simulink model "code_gen_man_bin"  (Simulink 7.5)
settings: Solver=FixedStepDiscrete  SolverMode=SingleTasking  StartTime=0.0  StopTime=10.0  FixedStep=0.01  RelTol=1e-3
InitFcn:
  | boat_constants
values from neighbouring files (symbols this model uses):
  figure8_waypoints = int32([ ... (first row only)    [boat_constants.m]
  InitialPoint = 0    [boat_constants.m]    (also in l2plus.m)
  IPStar = 0    [boat_constants.m]    (also in l2plus.m)
  ISA_g = 9.815    [boat_constants.m]
  MaxDwnPthStar = 1    [boat_constants.m]    (also in l2plus.m)
  OC2max = 49999    [boat_constants.m]    (also in simulation_constants.m)
  sampling_waypoints = int32([ ... (first row only)    [boat_constants.m]
  switchDistance = 4    [boat_constants.m]    (also in l2plus.m)
  T_step = 0.01    [boat_constants.m]    (also in common.m)
  tanIntercept = tan( 45*pi/180 )    [boat_constants.m]    (also in l2plus.m)
  test_waypoints = int32([ ... (first row only)    [boat_constants.m]
  TStar = single(4.5)    [boat_constants.m]    (also in l2plus.m = single(2))
  Turn2Track = 0    [boat_constants.m]    (also in l2plus.m)
  wheelbase = 3.27    [boat_constants.m]
undefined symbols (not defined in the file or in its folder): clearGpsData, clearSensorData, cpInitCommunications, DataEEInitAndClear, DataEEWrite, DiscIntNeverNeededParam, ecan1_buffered_transmit_matlab, ecan1_error_status_matlab, ecan1_init, GetAirData, getGpsData, getRevoData, getSensorData, GetThrottleData, GetWaterData, GetWindData, Init_onlyOnce, Init_Reset, initCalibrationRange, initGps, processNewCommData, processNewGpsData, processNewRevoData, setHilMode, u1, u2, uart1EnqueueStateData, uart2EnqueueActuatorData, y1
libraries: simulink x80, dsPICdrivers x50, uSimLib x4, simulink_need_slupdate x4
(part 5 of 6)

== system code_gen_man_bin/Controller/Radio Control Inputs1/Calibration/Update range from input1 ==
  note: Update lower range limit.
      | The new value is checked against a sane range of 5000-11000
      | to keep values realistic.
  note: Update upper range limit
  limitRange : Inport
  newValue : Inport  Port=2
  If : If  NumInputs=2  IfExpression=u1 < u2 & u1 > 5000 & u1 >= 0
  If Action Subsystem : Subsystem  TreatAsAtomicUnit=on
  If Action Subsystem1 : Subsystem  TreatAsAtomicUnit=on
  If Action Subsystem2 : Subsystem  TreatAsAtomicUnit=on
  If Action Subsystem3 : Subsystem  TreatAsAtomicUnit=on
  If1 : If  NumInputs=2  IfExpression=u1 > u2 & u1 < 11000 & u1 >= 0
  Merge : Merge
  Merge1 : Merge
  Mux : Mux  Inputs=2
  Selector : Selector  InputPortWidth=2  IndexOptions=Index vector (dialog)  Indices=[1]  OutputSizes=1
  Selector1 : Selector  InputPortWidth=2  IndexOptions=Index vector (dialog)  Indices=[2]  OutputSizes=1
  newRange : Outport
  wires:
  Selector/1 -> If/2, If Action Subsystem1/1(In1)
  Selector1/1 -> If Action Subsystem3/1(In1), If1/2
  Mux/1 -> newRange/1
  Merge1/1 -> Mux/2
  Merge/1 -> Mux/1
  If Action Subsystem3/1(Out1) -> Merge1/2
  If Action Subsystem2/1(Out1) -> Merge1/1
  If1/2 -> If Action Subsystem3/Action
  If1/1 -> If Action Subsystem2/Action
  If Action Subsystem1/1(Out1) -> Merge/2
  If Action Subsystem/1(Out1) -> Merge/1
  If/2 -> If Action Subsystem1/Action
  If/1 -> If Action Subsystem/Action
  newValue/1 -> If Action Subsystem/1(In1), If/1, If Action Subsystem2/1(In1), If1/1
  limitRange/1 -> Selector/1, Selector1/1

== system code_gen_man_bin/Controller/Radio Control Inputs1/Calibration/Update range from input2 ==
  note: Update lower range limit.
      | The new value is checked against a sane range of 5000-11000
      | to keep values realistic.
  note: Update upper range limit
  limitRange : Inport
  newValue : Inport  Port=2
  If : If  NumInputs=2  IfExpression=u1 < u2 & u1 > 5000 & u1 >= 0
  If Action Subsystem : Subsystem  TreatAsAtomicUnit=on
  If Action Subsystem1 : Subsystem  TreatAsAtomicUnit=on
  If Action Subsystem2 : Subsystem  TreatAsAtomicUnit=on
  If Action Subsystem3 : Subsystem  TreatAsAtomicUnit=on
  If1 : If  NumInputs=2  IfExpression=u1 > u2 & u1 < 11000 & u1 >= 0
  Merge : Merge
  Merge1 : Merge
  Mux : Mux  Inputs=2
  Selector : Selector  InputPortWidth=2  IndexOptions=Index vector (dialog)  Indices=[1]  OutputSizes=1
  Selector1 : Selector  InputPortWidth=2  IndexOptions=Index vector (dialog)  Indices=[2]  OutputSizes=1
  newRange : Outport
  wires:
  Selector/1 -> If/2, If Action Subsystem1/1(In1)
  Selector1/1 -> If Action Subsystem3/1(In1), If1/2
  Mux/1 -> newRange/1
  Merge1/1 -> Mux/2
  Merge/1 -> Mux/1
  If Action Subsystem3/1(Out1) -> Merge1/2
  If Action Subsystem2/1(Out1) -> Merge1/1
  If1/2 -> If Action Subsystem3/Action
  If1/1 -> If Action Subsystem2/Action
  If Action Subsystem1/1(Out1) -> Merge/2
  If Action Subsystem/1(Out1) -> Merge/1
  If/2 -> If Action Subsystem1/Action
  If/1 -> If Action Subsystem/Action
  newValue/1 -> If Action Subsystem/1(In1), If/1, If Action Subsystem2/1(In1), If1/1
  limitRange/1 -> Selector/1, Selector1/1

== system code_gen_man_bin/Controller/Radio Control Inputs1/Detect calibration trigger/State outputs ==
  note: Define state outputs:
      | State 0: Not in calibration mode
      |   - LED is off
      | State 1: Calibration mode trigger test
      |   - LED is blinking at 10Hz
      | State 2: Calibration mode
      |   - LED is on
  cState : Inport
  If Action Subsystem1 : Subsystem  TreatAsAtomicUnit=on
  If Action Subsystem2 : Subsystem  TreatAsAtomicUnit=on
  If Action Subsystem3 : Subsystem  TreatAsAtomicUnit=on
  If Action Subsystem4 : Subsystem  TreatAsAtomicUnit=on
  If1 : If  IfExpression=u1 == 0 | u1 == 3  ElseIfExpressions=u1 == 1 | u1 == 4, u1 == 2
  Merge : Merge  Inputs=4  InitialOutput=false
  Rate Transition : RateTransition
  Repeating Sequence Stair : simulink/Sources/Repeating Sequence Stair  SystemSampleTime=-1  OutValues=[1 0]  tsamp=.1  OutMin=[]  OutMax=[]  OutDataTypeStr=fixdt('boolean')  OutputDataTypeScalingMode=Specify via dialog  OutDataType=fixdt('boolean')  ConRadixGroup=Best Precision: Vector-wise  OutScaling=[]
  LED : Outport
  wires:
  cState/1 -> If1/1
  Merge/1 -> LED/1
  If1/1 -> If Action Subsystem1/Action
  If1/2 -> If Action Subsystem3/Action
  If Action Subsystem1/1(LED) -> Merge/1
  If Action Subsystem3/1(LED) -> Merge/2
  If1/4 -> If Action Subsystem2/Action
  If1/3 -> If Action Subsystem4/Action
  If Action Subsystem4/1(LED) -> Merge/3
  If Action Subsystem2/1(LED) -> Merge/4
  Repeating Sequence Stair/1 -> Rate Transition/1
  Rate Transition/1 -> If Action Subsystem3/1(Pulse)

== system code_gen_man_bin/Controller/Radio Control Inputs1/If Action Subsystem1/Add 8% center deadband ==
  In1 : Inport
  If : If  IfExpression=u1 > -36 & u1 < 36
  If Action Subsystem : Subsystem  TreatAsAtomicUnit=on
  If Action Subsystem1 : Subsystem  TreatAsAtomicUnit=on
  Merge : Merge
  Out1 : Outport
  wires:
  In1/1 -> If Action Subsystem/1(In1), If/1
  If/2 -> If Action Subsystem/Action
  If/1 -> If Action Subsystem1/Action
  If Action Subsystem/1(Out1) -> Merge/2
  If Action Subsystem1/1(Out1) -> Merge/1
  Merge/1 -> Out1/1

== system code_gen_man_bin/Controller/Radio Control Inputs1/If Action Subsystem3/Add 5% deadband about 0 ==
  In1 : Inport
  If : If  IfExpression=u1 < 43 & u1 > -43
  If Action Subsystem : Subsystem  TreatAsAtomicUnit=on
  If Action Subsystem1 : Subsystem  TreatAsAtomicUnit=on
  Merge : Merge
  Out1 : Outport
  wires:
  In1/1 -> If Action Subsystem/1(In1), If/1
  If/2 -> If Action Subsystem/Action
  If/1 -> If Action Subsystem1/Action
  If Action Subsystem1/1(Out1) -> Merge/1
  Merge/1 -> Out1/1
  If Action Subsystem/1(Out1) -> Merge/2

== system code_gen_man_bin/Controller/Radio Control Inputs1/If Action Subsystem5/Add 8% center deadband ==
  In1 : Inport
  If : If  IfExpression=u1 > 460 & u1 < 540
  If Action Subsystem : Subsystem  TreatAsAtomicUnit=on
  If Action Subsystem1 : Subsystem  TreatAsAtomicUnit=on
  Merge : Merge
  Out1 : Outport
  wires:
  In1/1 -> If Action Subsystem/1(In1), If/1
  If/2 -> If Action Subsystem/Action
  If/1 -> If Action Subsystem1/Action
  If Action Subsystem/1(Out1) -> Merge/2
  If Action Subsystem1/1(Out1) -> Merge/1
  Merge/1 -> Out1/1

== system code_gen_man_bin/Controller/Rudder sensor calibration/Throttle Command/Mux Everything ==
  reset : Inport  OutDataType=sfix(16)  OutScaling=2^0
  0x300 : Constant  Value=768  OutDataTypeMode=uint32  OutDataType=sfix(16)  OutScaling=2^0  OutDataTypeStr=uint32
  Data Type Conversion1 : DataTypeConversion  OutDataTypeMode=boolean  OutDataType=sfix(16)  OutScaling=2^0  OutDataTypeStr=boolean
  Data Type Conversion3 : DataTypeConversion  OutDataTypeMode=boolean  OutDataType=sfix(16)  OutScaling=2^0  OutDataTypeStr=boolean
  Detect Change : simulink/Logic and Bit Operations/Detect Change  SystemSampleTime=-1  vinit=0
  Detect Rise Positive : simulink/Logic and Bit Operations/Detect Rise Positive  SystemSampleTime=-1  vinit=0
  Disable motor : Constant  Value=[0 0 0 0 64 0]  OutDataTypeMode=uint8  OutDataType=sfix(16)  OutScaling=2^0  OutDataTypeStr=uint8
  Enable motor : Constant  Value=[0 0 0 0 32 0]  OutDataTypeMode=uint8  OutDataType=sfix(16)  OutScaling=2^0  OutDataTypeStr=uint8
  Message Length1 : Probe  ProbeSampleTime=off  ProbeComplexSignal=off  ProbeWidthDataType=uint8
  Switch : Switch  Criteria=u2 ~= 0  OutDataType=fixdt(1, 16)  OutScaling=2^0
  iden : Outport  OutDataType=sfix(16)  OutScaling=2^0
  data : Outport  Port=2  OutDataType=sfix(16)  OutScaling=2^0
  size : Outport  Port=3  OutDataType=sfix(16)  OutScaling=2^0
  trig : Outport  Port=4  OutDataType=sfix(16)  OutScaling=2^0
  wires:
  0x300/1 -> iden/1
  Message Length1/1 -> size/1
  Switch/1 -> data/1, Message Length1/1
  Disable motor/1 -> Switch/1
  Enable motor/1 -> Switch/3
  Data Type Conversion1/1 -> Switch/2
  Detect Rise Positive/1 -> Data Type Conversion1/1
  reset/1 -> Detect Rise Positive/1, Detect Change/1
  Detect Change/1 -> Data Type Conversion3/1
  Data Type Conversion3/1 -> trig/1

== system code_gen_man_bin/Controller/Split trackCommand to singular commands/Countdown timer for trigger/State transitions ==
  note: Define state transitions:
      | State 0: Not in calibration mode
      |   - Transition to state 1 if change
      | State 1: Transition trigger test
      |   - Transition to state 2 if level held
      |   - Transition to state 0 if level drops
      | State 2: Transition successful
      |   - Transition to state 0 if change
  timer : Inport
  level : Inport  Port=2
  timerState : Inport  Port=3
  If : If  NumInputs=3  IfExpression=u3 == 0 & u2 == 1  ElseIfExpressions=u3 == 1 & u2 == 0, u3 == 1 & u1 >= 100, u3 == 2 & u2 == 0
  Merge1 : Merge  Inputs=5  InitialOutput=false
  Merge2 : Merge  Inputs=5  InitialOutput=false
  Null transition (necessary for merge block) : Subsystem  TreatAsAtomicUnit=on
  Transition from 0 to 1 : Subsystem  TreatAsAtomicUnit=on
  Transition from 1 to 0 : Subsystem  TreatAsAtomicUnit=on
  Transition from 1 to 2 : Subsystem  TreatAsAtomicUnit=on
  Transition from 2 to 0 : Subsystem  TreatAsAtomicUnit=on
  startTimer : Outport
  trigger : Outport  Port=2
  wires:
  If/1 -> Transition from 0 to 1/Action
  If/5 -> Null transition (necessary for merge block)/Action
  timer/1 -> If/1
  timerState/1 -> If/3
  level/1 -> If/2
  If/2 -> Transition from 1 to 0/Action
  If/3 -> Transition from 1 to 2/Action
  If/4 -> Transition from 2 to 0/Action
  Merge1/1 -> startTimer/1
  Transition from 0 to 1/1(startTimer) -> Merge1/1
  Transition from 1 to 0/1(startTimer) -> Merge1/2
  Transition from 1 to 2/1(startTimer) -> Merge1/3
  Transition from 2 to 0/1(startTimer) -> Merge1/4
  Null transition (necessary for merge block)/1(startTimer) -> Merge1/5
  Merge2/1 -> trigger/1
  Transition from 0 to 1/2(trigger) -> Merge2/1
  Transition from 1 to 0/2(trigger) -> Merge2/2
  Transition from 1 to 2/2(trigger) -> Merge2/3
  Transition from 2 to 0/2(trigger) -> Merge2/4
  Null transition (necessary for merge block)/2(trigger) -> Merge2/5

== system code_gen_man_bin/Controller/Split trackCommand to singular commands/Countdown timer for trigger1/State transitions ==
  note: Define state transitions:
      | State 0: Not in calibration mode
      |   - Transition to state 1 if change
      | State 1: Transition trigger test
      |   - Transition to state 2 if level held
      |   - Transition to state 0 if level drops
      | State 2: Transition successful
      |   - Transition to state 0 if change
  timer : Inport
  level : Inport  Port=2
  timerState : Inport  Port=3
  If : If  NumInputs=3  IfExpression=u3 == 0 & u2 == 1  ElseIfExpressions=u3 == 1 & u2 == 0, u3 == 1 & u1 >= 100, u3 == 2 & u2 == 0
  Merge1 : Merge  Inputs=5  InitialOutput=false
  Merge2 : Merge  Inputs=5  InitialOutput=false
  Null transition (necessary for merge block) : Subsystem  TreatAsAtomicUnit=on
  Transition from 0 to 1 : Subsystem  TreatAsAtomicUnit=on
  Transition from 1 to 0 : Subsystem  TreatAsAtomicUnit=on
  Transition from 1 to 2 : Subsystem  TreatAsAtomicUnit=on
  Transition from 2 to 0 : Subsystem  TreatAsAtomicUnit=on
  startTimer : Outport
  trigger : Outport  Port=2
  wires:
  Null transition (necessary for merge block)/2(trigger) -> Merge2/5
  Transition from 2 to 0/2(trigger) -> Merge2/4
  Transition from 1 to 2/2(trigger) -> Merge2/3
  Transition from 1 to 0/2(trigger) -> Merge2/2
  Transition from 0 to 1/2(trigger) -> Merge2/1
  Merge2/1 -> trigger/1
  Null transition (necessary for merge block)/1(startTimer) -> Merge1/5
  Transition from 2 to 0/1(startTimer) -> Merge1/4
  Transition from 1 to 2/1(startTimer) -> Merge1/3
  Transition from 1 to 0/1(startTimer) -> Merge1/2
  Transition from 0 to 1/1(startTimer) -> Merge1/1
  Merge1/1 -> startTimer/1
  If/4 -> Transition from 2 to 0/Action
  If/3 -> Transition from 1 to 2/Action
  If/2 -> Transition from 1 to 0/Action
  level/1 -> If/2
  timerState/1 -> If/3
  timer/1 -> If/1
  If/5 -> Null transition (necessary for merge block)/Action
  If/1 -> Transition from 0 to 1/Action

== system code_gen_man_bin/Controller/Autonomous Controller/State Keeper & Estimator/GPS Estimator/Subsystem ==
  note: Multiply by .51444 to
      | convert knots to m/s
  gps : Inport
  Angle Conversion : uSimLib/Conversions/Angle Conversion  SystemSampleTime=-1  iu=deg  ou=rad
  Bus Selector : BusSelector  OutputSignals=sog
  Bus Selector1 : BusSelector  OutputSignals=cog
  Constant : Constant  Value=0  OutDataTypeMode=single  OutDataType=fixdt(1, 16)  OutScaling=2^0  OutDataTypeStr=single
  Gain : Gain  Gain=.5144444  ParameterDataType=fixdt(1, 16)  ParameterScaling=2^0  OutDataType=fixdt(1, 16)  OutScaling=2^0
  Mux : Mux  Inputs=3
  Product : Product  OutDataTypeMode=single  OutDataType=fixdt(1, 16)  OutScaling=2^0  OutDataTypeStr=single  RndMeth=Zero
  Product1 : Product  OutDataTypeMode=single  OutDataType=fixdt(1, 16)  OutScaling=2^0  OutDataTypeStr=single  RndMeth=Zero
  Reorder : Subsystem
  Trigonometric Function : Trigonometry
  Trigonometric Function1 : Trigonometry  Operator=cos
  velocity : Outport
  heading : Outport  Port=2
  pos : Outport  Port=3
  time : Outport  Port=4
  wires:
  Reorder/2(time) -> time/1
  Reorder/1(pos) -> pos/1
  Bus Selector/1 -> Gain/1  "<sog>"
  Angle Conversion/1 -> Trigonometric Function1/1, Trigonometric Function/1, heading/1
  Mux/1 -> velocity/1
  Constant/1 -> Mux/3
  Product/1 -> Mux/2
  Product1/1 -> Mux/1
  Trigonometric Function1/1 -> Product1/2
  Trigonometric Function/1 -> Product/2
  Bus Selector1/1 -> Angle Conversion/1  "<cog>"
  gps/1 -> Bus Selector1/1, Bus Selector/1, Reorder/1(In1)
  Gain/1 -> Product/1, Product1/1

== system code_gen_man_bin/Controller/Autonomous Controller/Throttle Command/Mux Everything/Build speed command ==
  CC : Inport  OutDataType=sfix(16)  OutScaling=2^0
  Constant : Constant  OutDataTypeMode=uint8  OutDataType=sfix(16)  OutScaling=2^0  OutDataTypeStr=uint8
  Constant1 : Constant  Value=0  OutDataTypeMode=uint8  OutDataType=sfix(16)  OutScaling=2^0  OutDataTypeStr=uint8
  Constant2 : Constant  Value=0  OutDataTypeMode=uint8  OutDataType=sfix(16)  OutScaling=2^0  OutDataTypeStr=uint8
  Constant3 : Constant  Value=5  OutDataTypeMode=uint8  OutDataType=sfix(16)  OutScaling=2^0  OutDataTypeStr=uint8
  Mux : Mux  Inputs=5
  uint16 to uchar : Subsystem  AncestorBlock=uSimLib/Conversions/uint16 to uchar
  msg : Outport  OutDataType=sfix(16)  OutScaling=2^0
  wires:
  CC/1 -> uint16 to uchar/1(ushort)
  Constant2/1 -> Mux/5
  Constant1/1 -> Mux/4
  Mux/1 -> msg/1
  Constant3/1 -> Mux/2
  Constant/1 -> Mux/1
  uint16 to uchar/1(uchar) -> Mux/3

== system code_gen_man_bin/Controller/RC Inputs/Map PWM values to Actuator Signals/Throttle Command/Mux Everything ==
  speed : Inport  OutDataType=sfix(16)  OutScaling=2^0
  enable : Inport  Port=2  OutDataType=sfix(16)  OutScaling=2^0
  Throttle : Inport  Port=3  OutDataType=sfix(16)  OutScaling=2^0
  0x300 : Constant  Value=768  OutDataTypeMode=uint32  OutDataType=sfix(16)  OutScaling=2^0  OutDataTypeStr=uint32
  0x301 : Constant  Value=769  OutDataTypeMode=uint32  OutDataType=sfix(16)  OutScaling=2^0  OutDataTypeStr=uint32
  Build speed command : Subsystem
  Enable motor : Constant  Value=[0 0 0 0 32 0]  OutDataTypeMode=uint8  OutDataType=sfix(16)  OutScaling=2^0  OutDataTypeStr=uint8
  Message Length1 : Probe  ProbeSampleTime=off  ProbeComplexSignal=off  ProbeWidthDataType=uint8
  Switch : Switch  Criteria=u2 ~= 0  Threshold=1
  Switch1 : Switch  Criteria=u2 ~= 0  OutDataType=fixdt(1, 16)  OutScaling=2^0
  iden : Outport  OutDataType=sfix(16)  OutScaling=2^0
  data : Outport  Port=2  OutDataType=sfix(16)  OutScaling=2^0
  size : Outport  Port=3  OutDataType=sfix(16)  OutScaling=2^0
  trig : Outport  Port=4  OutDataType=sfix(16)  OutScaling=2^0
  wires:
  Throttle/1 -> Build speed command/1(CC)
  Message Length1/1 -> size/1
  0x301/1 -> Switch/3
  Switch1/1 -> Message Length1/1, data/1
  0x300/1 -> Switch/1
  enable/1 -> Switch/2, Switch1/2
  speed/1 -> trig/1
  Enable motor/1 -> Switch1/1
  Build speed command/1(msg) -> Switch1/3
  Switch/1 -> iden/1

== system code_gen_man_bin/Controller/RC Inputs/Map PWM values to Actuator Signals/Throttle Command/Trigger Events ==
  Throttle : Inport  OutDataType=sfix(16)  OutScaling=2^0
  Data Type Conversion3 : DataTypeConversion  OutDataTypeMode=boolean  OutDataType=sfix(16)  OutScaling=2^0  OutDataTypeStr=boolean
  Detect Change : simulink/Logic and Bit Operations/Detect Change  SystemSampleTime=-1  vinit=0
  Shift Arithmetic : simulink/Logic and Bit Operations/Shift Arithmetic  SystemSampleTime=-1  nBitShiftRight=2  nBinPtShiftRight=0
  Weighted Moving Average : simulink_need_slupdate/Weighted Moving Average  mgainval=[.5 .5]  vinit=0.0  samptime=-1  OutDataTypeStr=Inherit: Inherit via back propagation  OutDataType=sfix(16)  OutScaling=2^-10  DoSatur=off  GainDataType=uint(16)  MatRadixGroup=Best Precision: Matrix-wise  GainScaling=2^-10
  Change Speed : Outport  OutDataType=sfix(16)  OutScaling=2^0
  wires:
  Throttle/1 -> Shift Arithmetic/1
  Detect Change/1 -> Data Type Conversion3/1
  Data Type Conversion3/1 -> Change Speed/1
  Weighted Moving Average/1 -> Detect Change/1
  Shift Arithmetic/1 -> Weighted Moving Average/1

== system code_gen_man_bin/Controller/Radio Control Inputs1/Calibration/Update range from input/If Action Subsystem ==
  In1 : Inport  OutDataType=fixdt(1, 16)  OutScaling=2^0
  Action Port : ActionPort  ActionType=then
  Out1 : Outport  OutDataType=fixdt(1, 16)  OutScaling=2^0
  wires:
  In1/1 -> Out1/1

== system code_gen_man_bin/Controller/Radio Control Inputs1/Calibration/Update range from input/If Action Subsystem1 ==
  In1 : Inport  OutDataType=fixdt(1, 16)  OutScaling=2^0
  Action Port : ActionPort  ActionType=else
  Out1 : Outport  OutDataType=fixdt(1, 16)  OutScaling=2^0
  wires:
  In1/1 -> Out1/1

== system code_gen_man_bin/Controller/Radio Control Inputs1/Calibration/Update range from input/If Action Subsystem2 ==
  In1 : Inport  OutDataType=fixdt(1, 16)  OutScaling=2^0
  Action Port : ActionPort  ActionType=then
  Out1 : Outport  OutDataType=fixdt(1, 16)  OutScaling=2^0
  wires:
  In1/1 -> Out1/1

== system code_gen_man_bin/Controller/Radio Control Inputs1/Calibration/Update range from input/If Action Subsystem3 ==
  In1 : Inport  OutDataType=fixdt(1, 16)  OutScaling=2^0
  Action Port : ActionPort  ActionType=else
  Out1 : Outport  OutDataType=fixdt(1, 16)  OutScaling=2^0
  wires:
  In1/1 -> Out1/1

== system code_gen_man_bin/Controller/Radio Control Inputs1/Calibration/Update range from input1/If Action Subsystem ==
  In1 : Inport  OutDataType=fixdt(1, 16)  OutScaling=2^0
  Action Port : ActionPort  ActionType=then
  Out1 : Outport  OutDataType=fixdt(1, 16)  OutScaling=2^0
  wires:
  In1/1 -> Out1/1

== system code_gen_man_bin/Controller/Radio Control Inputs1/Calibration/Update range from input1/If Action Subsystem1 ==
  In1 : Inport  OutDataType=fixdt(1, 16)  OutScaling=2^0
  Action Port : ActionPort  ActionType=else
  Out1 : Outport  OutDataType=fixdt(1, 16)  OutScaling=2^0
  wires:
  In1/1 -> Out1/1

== system code_gen_man_bin/Controller/Radio Control Inputs1/Calibration/Update range from input1/If Action Subsystem2 ==
  In1 : Inport  OutDataType=fixdt(1, 16)  OutScaling=2^0
  Action Port : ActionPort  ActionType=then
  Out1 : Outport  OutDataType=fixdt(1, 16)  OutScaling=2^0
  wires:
  In1/1 -> Out1/1

== system code_gen_man_bin/Controller/Radio Control Inputs1/Calibration/Update range from input1/If Action Subsystem3 ==
  In1 : Inport  OutDataType=fixdt(1, 16)  OutScaling=2^0
  Action Port : ActionPort  ActionType=else
  Out1 : Outport  OutDataType=fixdt(1, 16)  OutScaling=2^0
  wires:
  In1/1 -> Out1/1

== system code_gen_man_bin/Controller/Radio Control Inputs1/Calibration/Update range from input2/If Action Subsystem ==
  In1 : Inport  OutDataType=fixdt(1, 16)  OutScaling=2^0
  Action Port : ActionPort  ActionType=then
  Out1 : Outport  OutDataType=fixdt(1, 16)  OutScaling=2^0
  wires:
  In1/1 -> Out1/1

== system code_gen_man_bin/Controller/Radio Control Inputs1/Calibration/Update range from input2/If Action Subsystem1 ==
  In1 : Inport  OutDataType=fixdt(1, 16)  OutScaling=2^0
  Action Port : ActionPort  ActionType=else
  Out1 : Outport  OutDataType=fixdt(1, 16)  OutScaling=2^0
  wires:
  In1/1 -> Out1/1

== system code_gen_man_bin/Controller/Radio Control Inputs1/Calibration/Update range from input2/If Action Subsystem2 ==
  In1 : Inport  OutDataType=fixdt(1, 16)  OutScaling=2^0
  Action Port : ActionPort  ActionType=then
  Out1 : Outport  OutDataType=fixdt(1, 16)  OutScaling=2^0
  wires:
  In1/1 -> Out1/1

== system code_gen_man_bin/Controller/Radio Control Inputs1/Calibration/Update range from input2/If Action Subsystem3 ==
  In1 : Inport  OutDataType=fixdt(1, 16)  OutScaling=2^0
  Action Port : ActionPort  ActionType=else
  Out1 : Outport  OutDataType=fixdt(1, 16)  OutScaling=2^0
  wires:
  In1/1 -> Out1/1

== system code_gen_man_bin/Controller/Radio Control Inputs1/Detect calibration trigger/State outputs/If Action Subsystem1 ==
  Action Port : ActionPort  ActionType=then
  Constant1 : Constant  Value=false  OutDataType=fixdt(1, 16)  OutScaling=2^0  OutDataTypeStr=Inherit: Inherit via back propagation
  LED : Outport  OutDataType=fixdt(1, 16)  OutScaling=2^0  InitialOutput=false
  wires:
  Constant1/1 -> LED/1

== system code_gen_man_bin/Controller/Radio Control Inputs1/Detect calibration trigger/State outputs/If Action Subsystem2 ==
  Action Port : ActionPort  ActionType=else
  Constant1 : Constant  Value=false  OutDataType=fixdt(1, 16)  OutScaling=2^0  OutDataTypeStr=Inherit: Inherit via back propagation
  LED : Outport  OutDataType=fixdt(1, 16)  OutScaling=2^0  InitialOutput=false
  wires:
  Constant1/1 -> LED/1

== system code_gen_man_bin/Controller/Radio Control Inputs1/Detect calibration trigger/State outputs/If Action Subsystem3 ==
  Pulse : Inport
  Action Port : ActionPort  ActionType=elseif
  LED : Outport  OutDataType=fixdt(1, 16)  OutScaling=2^0  InitialOutput=false
  wires:
  Pulse/1 -> LED/1

== system code_gen_man_bin/Controller/Radio Control Inputs1/Detect calibration trigger/State outputs/If Action Subsystem4 ==
  Action Port : ActionPort  ActionType=elseif
  Constant1 : Constant  Value=true  OutDataType=fixdt(1, 16)  OutScaling=2^0  OutDataTypeStr=Inherit: Inherit via back propagation
  LED : Outport  OutDataType=fixdt(1, 16)  OutScaling=2^0  InitialOutput=false
  wires:
  Constant1/1 -> LED/1

== system code_gen_man_bin/Controller/Radio Control Inputs1/If Action Subsystem1/Add 8% center deadband/If Action Subsystem ==
  In1 : Inport  OutDataType=fixdt(1, 16)  OutScaling=2^0
  Action Port : ActionPort  ActionType=else
  Out1 : Outport  OutDataType=fixdt(1, 16)  OutScaling=2^0
  wires:
  In1/1 -> Out1/1

== system code_gen_man_bin/Controller/Radio Control Inputs1/If Action Subsystem1/Add 8% center deadband/If Action Subsystem1 ==
  Action Port : ActionPort  ActionType=then
  Constant : Constant  Value=0  OutDataType=fixdt(1, 16)  OutScaling=2^0  OutDataTypeStr=Inherit: Inherit via back propagation
  Out1 : Outport  OutDataType=fixdt(1, 16)  OutScaling=2^0  InitialOutput=50
  wires:
  Constant/1 -> Out1/1

== system code_gen_man_bin/Controller/Radio Control Inputs1/If Action Subsystem3/Add 5% deadband about 0/If Action Subsystem ==
  In1 : Inport  OutDataType=fixdt(1, 16)  OutScaling=2^0
  Action Port : ActionPort  ActionType=else
  Out1 : Outport  OutDataType=fixdt(1, 16)  OutScaling=2^0
  wires:
  In1/1 -> Out1/1

== system code_gen_man_bin/Controller/Radio Control Inputs1/If Action Subsystem3/Add 5% deadband about 0/If Action Subsystem1 ==
  Action Port : ActionPort  ActionType=then
  Constant : Constant  Value=0  OutDataType=fixdt(1, 16)  OutScaling=2^0  OutDataTypeStr=Inherit: Inherit via back propagation
  Out1 : Outport  OutDataType=fixdt(1, 16)  OutScaling=2^0  InitialOutput=0
  wires:
  Constant/1 -> Out1/1

== system code_gen_man_bin/Controller/Radio Control Inputs1/If Action Subsystem5/Add 8% center deadband/If Action Subsystem ==
  In1 : Inport  OutDataType=fixdt(1, 16)  OutScaling=2^0
  Action Port : ActionPort  ActionType=else
  Out1 : Outport  OutDataType=fixdt(1, 16)  OutScaling=2^0
  wires:
  In1/1 -> Out1/1

== system code_gen_man_bin/Controller/Radio Control Inputs1/If Action Subsystem5/Add 8% center deadband/If Action Subsystem1 ==
  Action Port : ActionPort  ActionType=then
  Constant : Constant  Value=500  OutDataType=fixdt(1, 16)  OutScaling=2^0  OutDataTypeStr=Inherit: Inherit via back propagation
  Out1 : Outport  OutDataType=fixdt(1, 16)  OutScaling=2^0  InitialOutput=50
  wires:
  Constant/1 -> Out1/1

== system code_gen_man_bin/Controller/Split trackCommand to singular commands/Countdown timer for trigger/State transitions/Null transition (necessary for merge block) ==
  Action Port : ActionPort  ActionType=else
  Constant1 : Constant  Value=false  OutDataTypeMode=boolean  OutDataType=fixdt(1, 16)  OutScaling=2^0  OutDataTypeStr=boolean
  Constant3 : Constant  Value=false  OutDataTypeMode=boolean  OutDataType=fixdt(1, 16)  OutScaling=2^0  OutDataTypeStr=boolean
  startTimer : Outport  OutDataType=fixdt(1, 16)  OutScaling=2^0  InitialOutput=false
  trigger : Outport  Port=2  OutDataType=fixdt(1, 16)  OutScaling=2^0  InitialOutput=false
  wires:
  Constant3/1 -> startTimer/1
  Constant1/1 -> trigger/1

== system code_gen_man_bin/Controller/Split trackCommand to singular commands/Countdown timer for trigger/State transitions/Transition from 0 to 1 ==
  Action Port : ActionPort  ActionType=then
  Constant : Constant  OutDataType=fixdt(1, 16)  OutScaling=2^0  OutDataTypeStr=Inherit: Inherit via back propagation
  Constant2 : Constant  Value=true  OutDataTypeMode=boolean  OutDataType=fixdt(1, 16)  OutScaling=2^0  OutDataTypeStr=boolean
  Constant3 : Constant  Value=false  OutDataTypeMode=boolean  OutDataType=fixdt(1, 16)  OutScaling=2^0  OutDataTypeStr=boolean
  Data Store Write : DataStoreWrite  DataStoreName=timerState  SampleTime=-1
  startTimer : Outport  OutDataType=fixdt(1, 16)  OutScaling=2^0  InitialOutput=true
  trigger : Outport  Port=2  OutDataType=fixdt(1, 16)  OutScaling=2^0  InitialOutput=true
  wires:
  Constant/1 -> Data Store Write/1
  Constant2/1 -> startTimer/1
  Constant3/1 -> trigger/1

== system code_gen_man_bin/Controller/Split trackCommand to singular commands/Countdown timer for trigger/State transitions/Transition from 1 to 0 ==
  Action Port : ActionPort  ActionType=elseif
  Constant : Constant  Value=0  OutDataType=fixdt(1, 16)  OutScaling=2^0  OutDataTypeStr=Inherit: Inherit via back propagation
  Constant1 : Constant  Value=false  OutDataTypeMode=boolean  OutDataType=fixdt(1, 16)  OutScaling=2^0  OutDataTypeStr=boolean
  Constant3 : Constant  Value=false  OutDataTypeMode=boolean  OutDataType=fixdt(1, 16)  OutScaling=2^0  OutDataTypeStr=boolean
  Data Store Write : DataStoreWrite  DataStoreName=timerState  SampleTime=-1
  startTimer : Outport  OutDataType=fixdt(1, 16)  OutScaling=2^0  InitialOutput=false
  trigger : Outport  Port=2  OutDataType=fixdt(1, 16)  OutScaling=2^0  InitialOutput=false
  wires:
  Constant/1 -> Data Store Write/1
  Constant3/1 -> startTimer/1
  Constant1/1 -> trigger/1

== system code_gen_man_bin/Controller/Split trackCommand to singular commands/Countdown timer for trigger/State transitions/Transition from 1 to 2 ==
  Action Port : ActionPort  ActionType=elseif
  Constant : Constant  Value=2  OutDataType=fixdt(1, 16)  OutScaling=2^0  OutDataTypeStr=Inherit: Inherit via back propagation
  Constant1 : Constant  Value=true  OutDataTypeMode=boolean  OutDataType=fixdt(1, 16)  OutScaling=2^0  OutDataTypeStr=boolean
  Constant3 : Constant  Value=false  OutDataTypeMode=boolean  OutDataType=fixdt(1, 16)  OutScaling=2^0  OutDataTypeStr=boolean
  Data Store Write : DataStoreWrite  DataStoreName=timerState  SampleTime=-1
  startTimer : Outport  OutDataType=fixdt(1, 16)  OutScaling=2^0  InitialOutput=false
  trigger : Outport  Port=2  OutDataType=fixdt(1, 16)  OutScaling=2^0  InitialOutput=false
  wires:
  Constant/1 -> Data Store Write/1
  Constant3/1 -> startTimer/1
  Constant1/1 -> trigger/1

== system code_gen_man_bin/Controller/Split trackCommand to singular commands/Countdown timer for trigger/State transitions/Transition from 2 to 0 ==
  Action Port : ActionPort  ActionType=elseif
  Constant : Constant  Value=0  OutDataType=fixdt(1, 16)  OutScaling=2^0  OutDataTypeStr=Inherit: Inherit via back propagation
  Constant1 : Constant  Value=false  OutDataTypeMode=boolean  OutDataType=fixdt(1, 16)  OutScaling=2^0  OutDataTypeStr=boolean
  Constant3 : Constant  Value=false  OutDataTypeMode=boolean  OutDataType=fixdt(1, 16)  OutScaling=2^0  OutDataTypeStr=boolean
  Data Store Write : DataStoreWrite  DataStoreName=timerState  SampleTime=-1
  startTimer : Outport  OutDataType=fixdt(1, 16)  OutScaling=2^0  InitialOutput=false
  trigger : Outport  Port=2  OutDataType=fixdt(1, 16)  OutScaling=2^0  InitialOutput=false
  wires:
  Constant/1 -> Data Store Write/1
  Constant3/1 -> startTimer/1
  Constant1/1 -> trigger/1

== system code_gen_man_bin/Controller/Split trackCommand to singular commands/Countdown timer for trigger1/State transitions/Null transition (necessary for merge block) ==
  Action Port : ActionPort  ActionType=else
  Constant1 : Constant  Value=false  OutDataTypeMode=boolean  OutDataType=fixdt(1, 16)  OutScaling=2^0  OutDataTypeStr=boolean
  Constant3 : Constant  Value=false  OutDataTypeMode=boolean  OutDataType=fixdt(1, 16)  OutScaling=2^0  OutDataTypeStr=boolean
  startTimer : Outport  OutDataType=fixdt(1, 16)  OutScaling=2^0  InitialOutput=false
  trigger : Outport  Port=2  OutDataType=fixdt(1, 16)  OutScaling=2^0  InitialOutput=false
  wires:
  Constant1/1 -> trigger/1
  Constant3/1 -> startTimer/1

== system code_gen_man_bin/Controller/Split trackCommand to singular commands/Countdown timer for trigger1/State transitions/Transition from 0 to 1 ==
  Action Port : ActionPort  ActionType=then
  Constant : Constant  OutDataType=fixdt(1, 16)  OutScaling=2^0  OutDataTypeStr=Inherit: Inherit via back propagation
  Constant2 : Constant  Value=true  OutDataTypeMode=boolean  OutDataType=fixdt(1, 16)  OutScaling=2^0  OutDataTypeStr=boolean
  Constant3 : Constant  Value=false  OutDataTypeMode=boolean  OutDataType=fixdt(1, 16)  OutScaling=2^0  OutDataTypeStr=boolean
  Data Store Write : DataStoreWrite  DataStoreName=timerState2  SampleTime=-1
  startTimer : Outport  OutDataType=fixdt(1, 16)  OutScaling=2^0  InitialOutput=true
  trigger : Outport  Port=2  OutDataType=fixdt(1, 16)  OutScaling=2^0  InitialOutput=true
  wires:
  Constant3/1 -> trigger/1
  Constant2/1 -> startTimer/1
  Constant/1 -> Data Store Write/1

== system code_gen_man_bin/Controller/Split trackCommand to singular commands/Countdown timer for trigger1/State transitions/Transition from 1 to 0 ==
  Action Port : ActionPort  ActionType=elseif
  Constant : Constant  Value=0  OutDataType=fixdt(1, 16)  OutScaling=2^0  OutDataTypeStr=Inherit: Inherit via back propagation
  Constant1 : Constant  Value=false  OutDataTypeMode=boolean  OutDataType=fixdt(1, 16)  OutScaling=2^0  OutDataTypeStr=boolean
  Constant3 : Constant  Value=false  OutDataTypeMode=boolean  OutDataType=fixdt(1, 16)  OutScaling=2^0  OutDataTypeStr=boolean
  Data Store Write : DataStoreWrite  DataStoreName=timerState2  SampleTime=-1
  startTimer : Outport  OutDataType=fixdt(1, 16)  OutScaling=2^0  InitialOutput=false
  trigger : Outport  Port=2  OutDataType=fixdt(1, 16)  OutScaling=2^0  InitialOutput=false
  wires:
  Constant1/1 -> trigger/1
  Constant3/1 -> startTimer/1
  Constant/1 -> Data Store Write/1

== system code_gen_man_bin/Controller/Split trackCommand to singular commands/Countdown timer for trigger1/State transitions/Transition from 1 to 2 ==
  Action Port : ActionPort  ActionType=elseif
  Constant : Constant  Value=2  OutDataType=fixdt(1, 16)  OutScaling=2^0  OutDataTypeStr=Inherit: Inherit via back propagation
  Constant1 : Constant  Value=true  OutDataTypeMode=boolean  OutDataType=fixdt(1, 16)  OutScaling=2^0  OutDataTypeStr=boolean
  Constant3 : Constant  Value=false  OutDataTypeMode=boolean  OutDataType=fixdt(1, 16)  OutScaling=2^0  OutDataTypeStr=boolean
  Data Store Write : DataStoreWrite  DataStoreName=timerState2  SampleTime=-1
  startTimer : Outport  OutDataType=fixdt(1, 16)  OutScaling=2^0  InitialOutput=false
  trigger : Outport  Port=2  OutDataType=fixdt(1, 16)  OutScaling=2^0  InitialOutput=false
  wires:
  Constant1/1 -> trigger/1
  Constant3/1 -> startTimer/1
  Constant/1 -> Data Store Write/1

== system code_gen_man_bin/Controller/Split trackCommand to singular commands/Countdown timer for trigger1/State transitions/Transition from 2 to 0 ==
  Action Port : ActionPort  ActionType=elseif
  Constant : Constant  Value=0  OutDataType=fixdt(1, 16)  OutScaling=2^0  OutDataTypeStr=Inherit: Inherit via back propagation
  Constant1 : Constant  Value=false  OutDataTypeMode=boolean  OutDataType=fixdt(1, 16)  OutScaling=2^0  OutDataTypeStr=boolean
  Constant3 : Constant  Value=false  OutDataTypeMode=boolean  OutDataType=fixdt(1, 16)  OutScaling=2^0  OutDataTypeStr=boolean
  Data Store Write : DataStoreWrite  DataStoreName=timerState2  SampleTime=-1
  startTimer : Outport  OutDataType=fixdt(1, 16)  OutScaling=2^0  InitialOutput=false
  trigger : Outport  Port=2  OutDataType=fixdt(1, 16)  OutScaling=2^0  InitialOutput=false
  wires:
  Constant1/1 -> trigger/1
  Constant3/1 -> startTimer/1
  Constant/1 -> Data Store Write/1

== system code_gen_man_bin/Controller/Autonomous Controller/State Keeper & Estimator/GPS Estimator/Subsystem/Reorder ==
  In1 : Inport
  Angle Conversion : uSimLib/Conversions/Angle Conversion  SystemSampleTime=-1  iu=deg  ou=rad
  Angle Conversion1 : uSimLib/Conversions/Angle Conversion  SystemSampleTime=-1  iu=deg  ou=rad
  Bias : Bias  Bias=2000
  Bus Selector : BusSelector  OutputSignals=latitude,longitude,year,month,day,hour,minute,second
  Constant : Constant  Value=0  OutDataTypeMode=single  OutDataType=fixdt(1, 16)  OutScaling=2^0  OutDataTypeStr=single
  Data Type Conversion{1..8} (8 alike) : DataTypeConversion  OutDataTypeMode=single  OutDataType=fixdt(1, 16)  OutScaling=2^0  OutDataTypeStr=single
  Mux : Mux  Inputs=7
  Mux1 : Mux  Inputs=3
  Phase shift2 : Constant  Value=-8  OutDataTypeMode=single  OutDataType=sfix(16)  OutScaling=2^0  OutDataTypeStr=single
  Scope : Scope
  pos : Outport
  time : Outport  Port=2
  wires:
  Data Type Conversion8/1 -> Angle Conversion/1
  Data Type Conversion7/1 -> Angle Conversion1/1
  Mux1/1 -> pos/1
  Constant/1 -> Mux1/3
  Angle Conversion1/1 -> Mux1/2
  Angle Conversion/1 -> Mux1/1, Scope/1
  Mux/1 -> time/1
  In1/1 -> Bus Selector/1
  Phase shift2/1 -> Mux/7
  Data Type Conversion6/1 -> Mux/6
  Data Type Conversion5/1 -> Mux/5
  Data Type Conversion4/1 -> Mux/4
  Data Type Conversion3/1 -> Mux/3
  Bus Selector/8 -> Data Type Conversion6/1  "<second>"
  Bus Selector/7 -> Data Type Conversion5/1  "<minute>"
  Bus Selector/6 -> Data Type Conversion4/1  "<hour>"
  Bus Selector/5 -> Data Type Conversion3/1  "<day>"
  Bus Selector/4 -> Data Type Conversion2/1  "<month>"
  Bus Selector/3 -> Data Type Conversion1/1  "<year>"
  Data Type Conversion2/1 -> Mux/2
  Bias/1 -> Mux/1
  Data Type Conversion1/1 -> Bias/1
  Bus Selector/2 -> Data Type Conversion7/1  "<longitude>"
  Bus Selector/1 -> Data Type Conversion8/1  "<latitude>"

== system code_gen_man_bin/Controller/Autonomous Controller/Throttle Command/Mux Everything/Build speed command/uint16 to uchar ==
  ushort : Inport
  Data Type Conversion : DataTypeConversion  OutDataTypeMode=uint16  OutDataType=fixdt(1, 16)  OutScaling=2^0  OutDataTypeStr=uint16  ConvertRealWorld=Stored Integer (SI)  RndMeth=Simplest
  Extract Bits1 : simulink/Logic and Bit Operations/Extract Bits  SystemSampleTime=-1  bitsToExtract=Upper half  numBits=8  bitIdxRange=[0 7]  outScalingMode=Treat bit field as an integer
  Extract Bits2 : simulink/Logic and Bit Operations/Extract Bits  SystemSampleTime=-1  bitsToExtract=Lower half  numBits=8  bitIdxRange=[0 7]  outScalingMode=Treat bit field as an integer
  Mux : Mux  Inputs=2
  uchar : Outport  OutDataType=fixdt(1, 16)  OutScaling=2^0
  wires:
  Data Type Conversion/1 -> Extract Bits2/1, Extract Bits1/1
  ushort/1 -> Data Type Conversion/1
  Extract Bits1/1 -> Mux/1
  Extract Bits2/1 -> Mux/2
  Mux/1 -> uchar/1

== system code_gen_man_bin/Controller/RC Inputs/Map PWM values to Actuator Signals/Throttle Command/Mux Everything/Build speed command ==
  CC : Inport  OutDataType=sfix(16)  OutScaling=2^0
  Constant : Constant  OutDataTypeMode=uint8  OutDataType=sfix(16)  OutScaling=2^0  OutDataTypeStr=uint8
  Constant1 : Constant  Value=0  OutDataTypeMode=uint8  OutDataType=sfix(16)  OutScaling=2^0  OutDataTypeStr=uint8
  Constant2 : Constant  Value=0  OutDataTypeMode=uint8  OutDataType=sfix(16)  OutScaling=2^0  OutDataTypeStr=uint8
  Constant3 : Constant  Value=5  OutDataTypeMode=uint8  OutDataType=sfix(16)  OutScaling=2^0  OutDataTypeStr=uint8
  Data Type Conversion1 : DataTypeConversion  OutDataTypeMode=uint8  OutDataType=sfix(16)  OutScaling=2^0  OutDataTypeStr=uint8  ConvertRealWorld=Stored Integer (SI)
  Data Type Conversion2 : DataTypeConversion  OutDataTypeMode=uint8  OutDataType=sfix(16)  OutScaling=2^0  OutDataTypeStr=uint8  ConvertRealWorld=Stored Integer (SI)
  Data Type Conversion3 : DataTypeConversion  OutDataTypeMode=uint16  OutDataType=sfix(16)  OutScaling=2^0  OutDataTypeStr=uint16  ConvertRealWorld=Stored Integer (SI)
  Extract Bits : simulink/Logic and Bit Operations/Extract Bits  SystemSampleTime=-1  bitsToExtract=Upper half  numBits=8  bitIdxRange=[24 31]  outScalingMode=Treat bit field as an integer
  Extract Bits1 : simulink/Logic and Bit Operations/Extract Bits  SystemSampleTime=-1  bitsToExtract=Lower half  numBits=8  bitIdxRange=[16 23]  outScalingMode=Treat bit field as an integer
  myMux : Stateflow chart  TreatAsAtomicUnit=on
  msg : Outport  OutDataType=sfix(16)  OutScaling=2^0
  wires:
  Constant2/1 -> myMux/6(u6)
  myMux/1(y) -> msg/1
  Constant3/1 -> myMux/2(u2)
  Constant/1 -> myMux/1(u1)
  Constant1/1 -> myMux/5(u5)
  Extract Bits1/1 -> Data Type Conversion2/1
  Extract Bits/1 -> Data Type Conversion1/1
  CC/1 -> Data Type Conversion3/1
  Data Type Conversion1/1 -> myMux/3(u3)
  Data Type Conversion2/1 -> myMux/4(u4)
  Data Type Conversion3/1 -> Extract Bits1/1, Extract Bits/1

== matlab function Controller/Autonomous Controller/State Keeper & Estimator/GPS Estimator/Calculate local position via velocity integral between true GPS updates ==
  data: latLonAlt input single size=[3 1]; localPosition output single; newData input boolean size=1; reset input boolean size=1; resetIntegrator output boolean size=1
function [localPosition,resetIntegrator] = estimateGPS(latLonAlt, newData, reset)
%#eml
% INPUTS:
% latLonAlt - the latitude, longitude, and altitude of the vehicle from GPS
% newData - A boolean signal specifying whether latLonAlt holds new data
% reset - A global reset boolean trigger.

% OUTPUTS:
% localPosition is the local position of the vehicle in relation to a recorded
% starting location in North-East-Down coordinates.
% resetIntegrator will reset the velocity integrator that's calculating the
% local position in between GPS reads.

persistent startingPosition lastKnownPosition newDataCounter;

% Reset everything on first startup or when a global reset is triggered
if isempty(startingPosition) || reset
    startingPosition = zeros(3, 1, 'single');
end
if isempty(lastKnownPosition) || reset
    lastKnownPosition = zeros(3, 1, 'single');
end
if isempty(newDataCounter) || reset
    newDataCounter = zeros(1, 1, 'uint8');
end

% Reset the integrator if a global reset is called
if reset
    resetIntegrator = true;
else
    resetIntegrator = false;
end

% Wait for 5 valid GPS inputs before latching a starting point
if newDataCounter < 5
    % Check that we have valid data before latching it.
    if newData && latLonAlt(1) ~= 0 && latLonAlt(2) ~= 0
        newDataCounter = newDataCounter + 1;
        startingPosition = latLonAlt;
    end
    
    % We output all 0s while we're waiting
    localPosition = zeros(3, 1, 'single');
else
    % Latch a new position if one's been received. Also reset the integrator
    % for this timestep as we have a "truth" position now.
    if newData
        lastKnownPosition = latLonAlt;
        resetIntegrator = true;
    end
    
    % Calculate the difference between the starting position and the last
    % known position.
    localPosition = dg2lg(startingPosition, latLonAlt);
end

% Not certain how this works or where I got it from.
function out = dg2lg(u1, u2)

dlat = (u2(1) - u1(1))*pi/180;
dlon = (u2(2) - u1(2))*pi/180;
lat = u1(1)*pi/180;
h = u2(3);
a = 6378137;
e2 = 0.00669437999014;

v=a./sqrt(1-e2.*sin(lat).^2);
r=v.*(1-e2)./(1-e2.*sin(lat).^2);
dx=dlat.*(r+h);
dy=dlon.*cos(lat).*(v+h);

% Map into North-East-Down coordinates
out = [dx; dy; 0];

== matlab function Sensor Inputs/RevoGS/Unpack sensor data ==
  data: heading output double; magStatus output double; pitch output double; pitchStatus output double; roll output double; rollStatus output double; dip output double; magneticMagnitude output double; newData output double; u input uint8
function [heading, magStatus, pitch, pitchStatus, roll, rollStatus, dip, magneticMagnitude, newData] = unpack(u)
%#eml

heading = typecast(u(1:4), 'single');
magStatus = u(5);
pitch = typecast(u(6:9), 'single');
pitchStatus = u(10);
roll = typecast(u(11:14), 'single');
rollStatus = u(15);
dip = typecast(u(16:19), 'single');
magneticMagnitude = typecast(u(20:21), 'uint16');
newData = u(22);

== matlab function Transmit actuator data/Package and Transmit Sensor Struct/Pack ==
  data: r_en input double; y output double; r_dir input double; r_up input double; r_per input double; b_en input double; b_dir input double; t_id input double; t_data input double; t_size input double; t_trig input double; time input double; rudderAngle input double; sensorOverride input double
function y = fcn(r_en, r_dir, r_up, r_per, b_en, b_dir, t_id, t_data, t_size, t_trig, time, rudderAngle, sensorOverride)
%#eml

y = zeros(27, 1, 'uint8');
y(1) = uint8(r_en);
y(2) = uint8(r_dir);
y(3) = uint8(bitand(r_up,hex2dec('FF')));
y(4) = uint8(bitand(bitshift(r_up,-8),hex2dec('FF')));
y(5) = uint8(bitand(r_per,hex2dec('FF')));
y(6) = uint8(bitand(bitshift(r_per,-8),hex2dec('FF')));
y(7) = uint8(b_en);
y(8) = uint8(b_dir);
y(9) = uint8(bitand(t_id,hex2dec('FF')));
y(10) = uint8(bitand(bitshift(t_id,-8),hex2dec('FF')));
y(11) = uint8(bitand(bitshift(t_id,-16),hex2dec('FF')));
y(12) = uint8(bitand(bitshift(t_id,-24),hex2dec('FF')));
y(13:18) = t_data(1:6);
y(19) = t_size;
y(20) = uint8(t_trig);
y(21) = uint8(bitand(typecast(time,'uint16'),hex2dec('FF')));
y(22) = uint8(bitand(bitshift(typecast(time,'uint16'),-8),hex2dec('FF')));
y(23) = uint8(bitand(typecast(rudderAngle,'uint32'),hex2dec('FF')));
y(24) = uint8(bitand(bitshift(typecast(rudderAngle,'uint32'),-8),hex2dec('FF')));
y(25) = uint8(bitand(bitshift(typecast(rudderAngle,'uint32'),-16),hex2dec('FF')));
y(26) = uint8(bitand(bitshift(typecast(rudderAngle,'uint32'),-24),hex2dec('FF')));
y(27) = sensorOverride

== matlab function Transmit actuator data/Package and Transmit Sensor Struct/Build HIL sentence/Pack ==
  data: a input double; y output double; b input double; c input double; d input double; e input double; f input double
function y = fcn(a, b, c, d, e, f)
%#eml

y = zeros(34, 1, 'uint8');
y(1) = a;
y(2) = b;
y(3:31) = c;
y(32) = d;
y(33) = e;
y(34) = f;

== matlab function Controller/RC Inputs/Map PWM values to Actuator Signals/Throttle Command/Mux Everything/Build speed command/myMux ==
  data: u1 input double; y output double; u2 input double; u3 input double; u4 input double; u5 input double; u6 input double
function y = myMux(u1, u2, u3, u4, u5, u6)
y = [u1(1); u2(1); u3(1); u4(1); u5(1); u6(1);];

== matlab function Sensor Inputs/Parse for HIL data/Unpack sensor data ==
  data: u input uint8; throttle output double; latitude output double; longitude output double; altitude output double; year output double; month output double; day output double; hour output double; minute output double; second output double; cog output double; sog output double; newGpsData output double; rudderPosition output double; rudderStarboardLimit output double; rudderPortLimit output double; ballastPosition output double; ballastStarboardLimit output double; ballastPortLimit output double; timestamp output double; newData output double
function [throttle, latitude, longitude, altitude, year, month, day, hour, minute, second, cog, sog, newGpsData, rudderPosition, rudderStarboardLimit, rudderPortLimit, ballastPosition, ballastStarboardLimit, ballastPortLimit, timestamp, newData] = unpack(u)
%#eml

throttle = typecast(u(1:2), 'int16');
latitude = typecast(u(3:6), 'single');
longitude = typecast(u(7:10), 'single');
altitude = typecast(u(11:14), 'single');
year = u(15);
month = u(16);
day = u(17);
hour = u(18);
minute = u(19);
second = u(20);
cog = typecast(u(21:24), 'single');
sog = typecast(u(25:28), 'single');
newGpsData = u(29);
rudderPosition = typecast(u(30:31), 'uint16');
rudderStarboardLimit = u(32);
rudderPortLimit = u(33);
ballastPosition = typecast(u(34:35), 'uint16');
ballastStarboardLimit = u(36);
ballastPortLimit = u(37);
timestamp = typecast(u(38:39), 'int16');
newData = u(40);
